simulink model "SEIR_model"  (R2019b)
settings: Solver=VariableStepAuto  StartTime=0.0  StopTime=1000  RelTol=1e-3
undefined symbols (not defined in the file): beta, epsilon, gamma, I0, mu, p, r, R0, S0
settings Model: Creator=64546  LastModifiedBy=64546

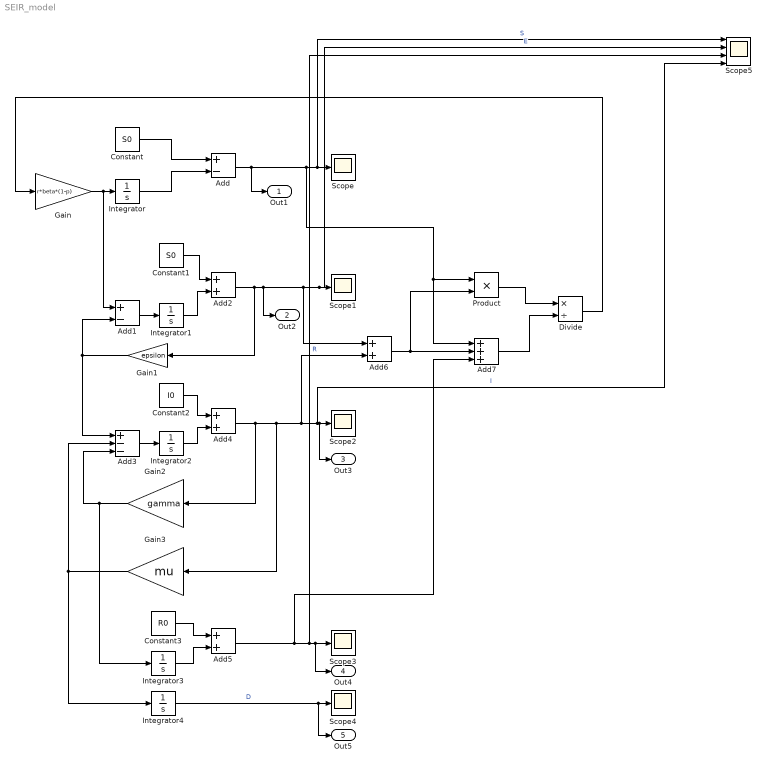
== system SEIR_model ==
  Add : Sum  Inputs=+-
  Add1 : Sum  Inputs=+-
  Add{2,4..6} (4 alike) : Sum
  Add3 : Sum  Inputs=+--
  Add7 : Sum  Inputs=+++
  Constant : Constant  Value=S0
  Constant1 : Constant  Value=S0
  Constant2 : Constant  Value=I0
  Constant3 : Constant  Value=R0
  Divide : Product  Inputs=*/
  Gain : Gain  Gain=r*beta*(1-p)
  Gain1 : Gain  Gain=epsilon
  Gain2 : Gain  Gain=gamma
  Gain3 : Gain  Gain=mu
  Integrator{,1..4} (5 alike) : Integrator
  Product : Product
  Scope{,1..4} (5 alike) : Scope
  Scope5 : Scope  NumInputPorts=4
  Out1 : Outport
  Out2 : Outport  Port=2
  Out3 : Outport  Port=3
  Out4 : Outport  Port=4
  Out5 : Outport  Port=5
  wires:
  Constant/1 -> Add/1
  Integrator/1 -> Add/2
  Gain/1 -> Add1/1, Integrator/1
  Add/1 -> Out1/1, Product/1, Add7/1, Scope5/1, Scope/1  "S"
  Gain1/1 -> Add1/2, Add3/1
  Add1/1 -> Integrator1/1
  Constant1/1 -> Add2/1
  Integrator1/1 -> Add2/2
  Add2/1 -> Gain1/1, Out2/1, Add6/1, Scope5/2, Scope1/1  "E"
  Gain2/1 -> Integrator3/1, Add3/3
  Add3/1 -> Integrator2/1
  Constant2/1 -> Add4/1
  Integrator2/1 -> Add4/2
  Add4/1 -> Gain2/1, Gain3/1, Add6/2, Scope5/4, Out3/1, Scope2/1  "I"
  Gain3/1 -> Integrator4/1, Add3/2
  Constant3/1 -> Add5/1
  Integrator3/1 -> Add5/2
  Add5/1 -> Add7/3, Scope5/3, Out4/1, Scope3/1  "R"
  Integrator4/1 -> Out5/1, Scope4/1  "D"
  Add6/1 -> Product/2, Add7/2
  Product/1 -> Divide/1
  Add7/1 -> Divide/2
  Divide/1 -> Gain/1
